simulink library "inp"  (R2021b)
settings: Solver=VariableStepAuto  StartTime=0.0  StopTime=10.0  RelTol=1e-3
undefined symbols (not defined in the file): C_TASK_5MS_S, FALSE, KINP_AcoreReadyToSlp_flg_ovrdflg, KINP_AcoreReadyToSlp_flg_ovrdval, KINP_AllowMovThd_OTA_enum_ovrdflg, KINP_AllowMovThd_OTA_enum_ovrdval, KINP_APSAngleTarget_Deg_ovrdflg, KINP_APSAngleTarget_Deg_ovrdval, KINP_APSDecReq_mps2_ovrdflg, KINP_APSDecReq_mps2_ovrdval, KINP_APSDecReqA_flg_ovrdflg, KINP_APSDecReqA_flg_ovrdval, KINP_APSDFLL_cm_ovrdflg, KINP_APSDFLL_cm_ovrdval, KINP_APSDFLR_cm_ovrdflg, KINP_APSDFLR_cm_ovrdval, KINP_APSDRLL_cm_ovrdflg, KINP_APSDRLL_cm_ovrdval, KINP_APSDRLR_cm_ovrdflg, KINP_APSDRLR_cm_ovrdval, KINP_APSExitCondition_enum_ovrdflg, KINP_APSExitCondition_enum_ovrdval, KINP_APSHWVer_enum_ovrdflg, KINP_APSHWVer_enum_ovrdval, KINP_APSProgressPCT_pct_ovrdflg, KINP_APSProgressPCT_pct_ovrdval, KINP_APSReq_enum_ovrdflg, KINP_APSReq_enum_ovrdval, KINP_APSRQDisplay_enum_ovrdflg, KINP_APSRQDisplay_enum_ovrdval, KINP_APSRqEPASCtrl_flg_ovrdflg, KINP_APSRqEPASCtrl_flg_ovrdval, KINP_APSShiftPosnReq_enum_ovrdval, KINP_APSShiftPosnReq_enum_ovrflg, KINP_APSSpeedCMD_kph_ovrdval, KINP_APSSpeedCMD_kph_ovrflg, KINP_APSStaSystem_enum_ovrdflg, KINP_APSStaSystem_enum_ovrdval, KINP_APSSWVer_enum_ovrdflg, KINP_APSSWVer_enum_ovrdval, KINP_APSVMCReqA_flg_ovrdval, KINP_APSVMCReqA_flg_ovrflg, KINP_APSVRqEPASCtrl_flg_ovrdflg, KINP_APSVRqEPASCtrl_flg_ovrdval, KINP_AuxBattVolmV_mV_ovrdflg, KINP_AuxBattVolmV_mV_ovrdval, KINP_CAASSta_enum_ovrdflg, KINP_CAASSta_enum_ovrdval, KINP_CAASVMCReqA_flg_ovrdval, KINP_CAASVMCReqA_flg_ovrflg, KINP_Chime_enum_ovrdflg, KINP_Chime_enum_ovrdval, KINP_ClearDTCcmd_flg_ovrdflg, KINP_ClearDTCcmd_flg_ovrdval, KINP_EvccAplusPwrUpReq_flg_ovrdflg, KINP_EvccAplusPwrUpReq_flg_ovrdval, KINP_LFID_raw_ovrdval, KINP_LFID_raw_ovrflg, KINP_LRID_raw_ovrdval, KINP_MemOffsetAccX_raw16_ovrdflg ... (+118)
libraries: FVT_lib x503, hcu_lib x1
(part 4 of 16)

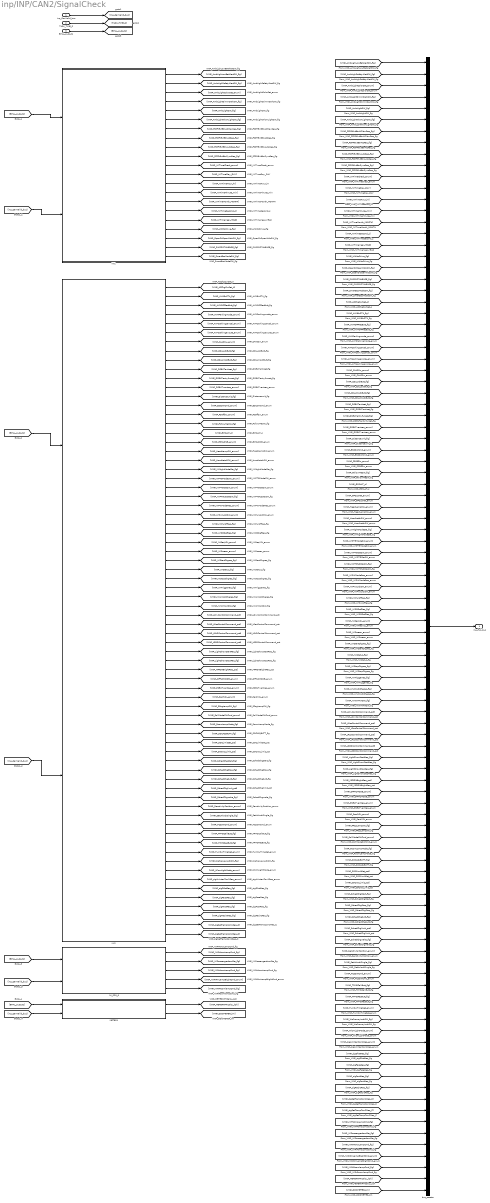
== system inp/INP/CAN2/SignalCheck ==
  inp_CanValid_bus : Inport
  TASK_TIME_S : Inport  Port=2
  BHAL_outputs : Inport  Port=3
  IVI1 : Subsystem
  IVI2 : Subsystem
  IVI_P20_0 : Subsystem
  METER1 : Subsystem
  bus_creator : BusCreator  Inputs=100
  inp_Hal_bus : Outport
  wires:
  inp_CanValid_bus/1 -> [inp_CanValid_bus]
  TASK_TIME_S/1 -> [TASK_TIME_S]
  BHAL_outputs/1 -> [BHAL_outputs]
  [BHAL_outputs] -> IVI1/1(BHAL_outputs)
  [inp_CanValid_bus] -> IVI1/2(inp_CanValid_bus)
  IVI1/1(VINP_AmbLighLowBatAlertSW_flg) -> [VINP_AmbLighLowBatAlertSW_flg]
  IVI1/2(VINP_AmbLighSafetyAlertSW_flg) -> [VINP_AmbLighSafetyAlertSW_flg]
  IVI1/3(VINP_AmbLightColorSet_enum) -> [VINP_AmbLightColorSet_enum]
  IVI1/4(VINP_AmbLightDimInDarkSW_flg) -> [VINP_AmbLightDimInDarkSW_flg]
  IVI1/5(VINP_AmbLightSW_flg) -> [VINP_AmbLightSW_flg]
  IVI1/6(VINP_AmbLightWlcmLightSW_flg) -> [VINP_AmbLightWlcmLightSW_flg]
  IVI1/7(VINP_FCPFrEvtBtnACMaxReq_flg) -> [VINP_FCPFrEvtBtnACMaxReq_flg]
  IVI1/8(VINP_FCPFrEvtBtnACReq_flg) -> [VINP_FCPFrEvtBtnACReq_flg]
  IVI1/9(VINP_FCPFrEvtBtnAutoReq_flg) -> [VINP_FCPFrEvtBtnAutoReq_flg]
  IVI1/10(VINP_FCPFrEvtBtnSyncReq_flg) -> [VINP_FCPFrEvtBtnSyncReq_flg]
  IVI1/11(VINP_IVITimeCheck_enum) -> [VINP_IVITimeCheck_enum]
  IVI1/12(VINP_IVITimeDay_DAY) -> [VINP_IVITimeDay_DAY]
  IVI1/13(VINP_IVITimeHour_hr) -> [VINP_IVITimeHour_hr]
  IVI1/14(VINP_IVITimeMinute_min) -> [VINP_IVITimeMinute_min]
  IVI1/15(VINP_IVITimeMonth_MONTH) -> [VINP_IVITimeMonth_MONTH]
  IVI1/16(VINP_IVITimeSecond_s) -> [VINP_IVITimeSecond_s]
  IVI1/17(VINP_IVITimeYear_YEAR) -> [VINP_IVITimeYear_YEAR]
  IVI1/18(VINP_LINKtoDrive_flg) -> [VINP_LINKtoDrive_flg]
  IVI1/19(VINP_OpenDrOpenWdoSW_flg) -> [VINP_OpenDrOpenWdoSW_flg]
  IVI1/20(VINP_PWCONTINUEUSE_flg) -> [VINP_PWCONTINUEUSE_flg]
  IVI1/21(VINP_SmartEcoModeSW_flg) -> [VINP_SmartEcoModeSW_flg]
  [BHAL_outputs] -> IVI2/1(BHAL_outputs)
  [inp_CanValid_bus] -> IVI2/2(inp_CanValid_bus)
  IVI2/1(VINP_ACChgCurSet_A) -> [VINP_ACChgCurSet_A]
  IVI2/2(VINP_AVMErrSTA_flg) -> [VINP_AVMErrSTA_flg]
  IVI2/3(VINP_AVMOFFRecButt_flg) -> [VINP_AVMOFFRecButt_flg]
  IVI2/4(VINP_AVMParkingmode_enum) -> [VINP_AVMParkingmode_enum]
  IVI2/5(VINP_AVMparkingcancel_enum) -> [VINP_AVMparkingcancel_enum]
  IVI2/6(VINP_AVMparkingexcute_enum) -> [VINP_AVMparkingexcute_enum]
  IVI2/7(VINP_CAASSw_enum) -> [VINP_CAASSw_enum]
  IVI2/8(VINP_CDLLockButt_flg) -> [VINP_CDLLockButt_flg]
  IVI2/9(VINP_CDLUnlockButt_flg) -> [VINP_CDLUnlockButt_flg]
  IVI2/10(VINP_DSEATantiset_flg) -> [VINP_DSEATantiset_flg]
  IVI2/11(VINP_DSEATentryfunset_flg) -> [VINP_DSEATentryfunset_flg]
  IVI2/12(VINP_DSEATventreq_enum) -> [VINP_DSEATventreq_enum]
  IVI2/13(VINP_Distanceunit_flg) -> [VINP_Distanceunit_flg]
  IVI2/14(VINP_ESCSWCmd_enum) -> [VINP_ESCSWCmd_enum]
  IVI2/15(VINP_FSOffSw_enum) -> [VINP_FSOffSw_enum]
  IVI2/16(VINP_FollowMeSW_flg) -> [VINP_FollowMeSW_flg]
  IVI2/17(VINP_GPSLAT_s) -> [VINP_GPSLAT_s]
  IVI2/18(VINP_GPSLONG_enum) -> [VINP_GPSLONG_enum]
  IVI2/19(VINP_HeadLampSW_enum) -> [VINP_HeadLampSW_enum]
  IVI2/20(VINP_HoodLatchSW_enum) -> [VINP_HoodLatchSW_enum]
  IVI2/21(VINP_IVINightModeSta_flg) -> [VINP_IVINightModeSta_flg]
  IVI2/22(VINP_IVIPTGModeSW_enum) -> [VINP_IVIPTGModeSW_enum]
  IVI2/23(VINP_IVIPTGStaSW_enum) -> [VINP_IVIPTGStaSW_enum]
  IVI2/24(VINP_IVIPTGUSStaSW_flg) -> [VINP_IVIPTGUSStaSW_flg]
  IVI2/25(VINP_IVIPWModeReq_enum) -> [VINP_IVIPWModeReq_enum]
  IVI2/26(VINP_IVIPwrLockSW_enum) -> [VINP_IVIPwrLockSW_enum]
  IVI2/27(VINP_IVIPwroffreq_flg) -> [VINP_IVIPwroffreq_flg]
  IVI2/28(VINP_IVIRRDefReq_flg) -> [VINP_IVIRRDefReq_flg]
  IVI2/29(VINP_IVIReqV2L_enum) -> [VINP_IVIReqV2L_enum]
  IVI2/30(VINP_IVIScreen_enum) -> [VINP_IVIScreen_enum]
  IVI2/31(VINP_IVIStartChgreq_flg) -> [VINP_IVIStartChgreq_flg]
  IVI2/32(VINP_IVIStatus_flg) -> [VINP_IVIStatus_flg]
  IVI2/33(VINP_IVIStopChgreq_flg) -> [VINP_IVIStopChgreq_flg]
  IVI2/34(VINP_IVITriggerreq_flg) -> [VINP_IVITriggerreq_flg]
  IVI2/35(VINP_IVIUnlockChgreq_flg) -> [VINP_IVIUnlockChgreq_flg]
  IVI2/36(VINP_IVIWIMAINSW_flg) -> [VINP_IVIWIMAINSW_flg]
  IVI2/37(VINP_LDrvControlCommand_pct) -> [VINP_LDrvControlCommand_pct]
  IVI2/38(VINP_LPasControlCommand_pct) -> [VINP_LPasControlCommand_pct]
  IVI2/39(VINP_LRLDControlCommand_pct) -> [VINP_LRLDControlCommand_pct]
  IVI2/40(VINP_LRRDControlCommand_pct) -> [VINP_LRRDControlCommand_pct]
  IVI2/41(VINP_LightShowStartReq_flg) -> [VINP_LightShowStartReq_flg]
  IVI2/42(VINP_LightShowStopReq_flg) -> [VINP_LightShowStopReq_flg]
  IVI2/43(VINP_MFRDNBrightReq_pct) -> [VINP_MFRDNBrightReq_pct]
  IVI2/44(VINP_OFFACMODE_enum) -> [VINP_OFFACMODE_enum]
  IVI2/45(VINP_PSEATventreq_enum) -> [VINP_PSEATventreq_enum]
  IVI2/46(VINP_PerdV2L_enum) -> [VINP_PerdV2L_enum]
  IVI2/47(VINP_RFogLampSW_flg) -> [VINP_RFogLampSW_flg]
  IVI2/48(VINP_RollModeSWCmd_enum) -> [VINP_RollModeSWCmd_enum]
  IVI2/49(VINP_RoomLampMode_flg) -> [VINP_RoomLampMode_flg]
  IVI2/50(VINP_SOCADJBUTT_flg) -> [VINP_SOCADJBUTT_flg]
  IVI2/51(VINP_SOCLimitSet_pct) -> [VINP_SOCLimitSet_pct]
  IVI2/52(VINP_SOCV2LLimit_pct) -> [VINP_SOCV2LLimit_pct]
  IVI2/53(VINP_SchedChgStart_flg) -> [VINP_SchedChgStart_flg]
  IVI2/54(VINP_SchedChgStop_flg) -> [VINP_SchedChgStop_flg]
  IVI2/55(VINP_SchedChgbutt_flg) -> [VINP_SchedChgbutt_flg]
  IVI2/56(VINP_SchedChglimit_pct) -> [VINP_SchedChglimit_pct]
  IVI2/57(VINP_SchedChgwake_flg) -> [VINP_SchedChgwake_flg]
  IVI2/58(VINP_SenstivityPosition_enum) -> [VINP_SenstivityPosition_enum]
  IVI2/59(VINP_SetUnlockSingle_flg) -> [VINP_SetUnlockSingle_flg]
  IVI2/60(VINP_TCSSWCmd_enum) -> [VINP_TCSSWCmd_enum]
  IVI2/61(VINP_TPMSCaliButt_flg) -> [VINP_TPMSCaliButt_flg]
  IVI2/62(VINP_TPMSResButt_flg) -> [VINP_TPMSResButt_flg]
  IVI2/63(VINP_TurnSwTimeSet_enum) -> [VINP_TurnSwTimeSet_enum]
  IVI2/64(VINP_WalkawayLockSW_flg) -> [VINP_WalkawayLockSW_flg]
  IVI2/65(VINP_WlcmLightMode_enum) -> [VINP_WlcmLightMode_enum]
  IVI2/66(VINP_sigAirIntenZon1Req_enum) -> [VINP_sigAirIntenZon1Req_enum]
  IVI2/67(VINP_sigDfrstReq_flg) -> [VINP_sigDfrstReq_flg]
  IVI2/68(VINP_sigFaceReq_flg) -> [VINP_sigFaceReq_flg]
  IVI2/69(VINP_sigFootReq_flg) -> [VINP_sigFootReq_flg]
  IVI2/70(VINP_sigRecircReq_flg) -> [VINP_sigRecircReq_flg]
  IVI2/71(VINP_sigSetTempZon1Req_C) -> [VINP_sigSetTempZon1Req_C]
  IVI2/72(VINP_sigSetTempZon2Req_C) -> [VINP_sigSetTempZon2Req_C]
  [BHAL_outputs] -> IVI_P20_0/1(BHAL_outputs)
  [inp_CanValid_bus] -> IVI_P20_0/2(inp_CanValid_bus)
  IVI_P20_0/1(VINP_IVIFrAtmoLampCmd_flg) -> [VINP_IVIFrAtmoLampCmd_flg]
  IVI_P20_0/2(VINP_IVIPassengerdoorSta_flg) -> [VINP_IVIPassengerdoorSta_flg]
  IVI_P20_0/3(VINP_IVIRrAtmoLampCmd_flg) -> [VINP_IVIRrAtmoLampCmd_flg]
  IVI_P20_0/4(VINP_IVIRrRmLampBrightCmd_enum) -> [VINP_IVIRrRmLampBrightCmd_enum]
  IVI_P20_0/5(VINP_IVIRrRoomlampCmd_flg) -> [VINP_IVIRrRoomlampCmd_flg]
  [BHAL_outputs] -> METER1/1(BHAL_outputs)
  [inp_CanValid_bus] -> METER1/2(inp_CanValid_bus)
  METER1/1(VINP_METERKPHCalcu_kph) -> [VINP_METERKPHCalcu_kph]
  METER1/2(VINP_ODOMETER_km) -> [VINP_ODOMETER_km]
  bus_creator/1 -> inp_Hal_bus/1
  [VINP_AmbLighLowBatAlertSW_flg] -> bus_creator/1
  [VINP_AmbLighSafetyAlertSW_flg] -> bus_creator/2
  [VINP_AmbLightColorSet_enum] -> bus_creator/3
  [VINP_AmbLightDimInDarkSW_flg] -> bus_creator/4
  [VINP_AmbLightSW_flg] -> bus_creator/5
  [VINP_AmbLightWlcmLightSW_flg] -> bus_creator/6
  [VINP_FCPFrEvtBtnACMaxReq_flg] -> bus_creator/7
  [VINP_FCPFrEvtBtnACReq_flg] -> bus_creator/8
  [VINP_FCPFrEvtBtnAutoReq_flg] -> bus_creator/9
  [VINP_FCPFrEvtBtnSyncReq_flg] -> bus_creator/10
  [VINP_IVITimeCheck_enum] -> bus_creator/11
  [VINP_IVITimeDay_DAY] -> bus_creator/12
  [VINP_IVITimeHour_hr] -> bus_creator/13
  [VINP_IVITimeMinute_min] -> bus_creator/14
  [VINP_IVITimeMonth_MONTH] -> bus_creator/15
  [VINP_IVITimeSecond_s] -> bus_creator/16
  [VINP_IVITimeYear_YEAR] -> bus_creator/17
  [VINP_LINKtoDrive_flg] -> bus_creator/18
  [VINP_OpenDrOpenWdoSW_flg] -> bus_creator/19
  [VINP_PWCONTINUEUSE_flg] -> bus_creator/20
  [VINP_SmartEcoModeSW_flg] -> bus_creator/21
  [VINP_ACChgCurSet_A] -> bus_creator/22
  [VINP_AVMErrSTA_flg] -> bus_creator/23
  [VINP_AVMOFFRecButt_flg] -> bus_creator/24
  [VINP_AVMParkingmode_enum] -> bus_creator/25
  [VINP_AVMparkingcancel_enum] -> bus_creator/26
  [VINP_AVMparkingexcute_enum] -> bus_creator/27
  [VINP_CAASSw_enum] -> bus_creator/28
  [VINP_CDLLockButt_flg] -> bus_creator/29
  [VINP_CDLUnlockButt_flg] -> bus_creator/30
  [VINP_DSEATantiset_flg] -> bus_creator/31
  [VINP_DSEATentryfunset_flg] -> bus_creator/32
  [VINP_DSEATventreq_enum] -> bus_creator/33
  [VINP_Distanceunit_flg] -> bus_creator/34
  [VINP_ESCSWCmd_enum] -> bus_creator/35
  [VINP_FSOffSw_enum] -> bus_creator/36
  [VINP_FollowMeSW_flg] -> bus_creator/37
  [VINP_GPSLAT_s] -> bus_creator/38
  [VINP_GPSLONG_enum] -> bus_creator/39
  [VINP_HeadLampSW_enum] -> bus_creator/40
  [VINP_HoodLatchSW_enum] -> bus_creator/41
  [VINP_IVINightModeSta_flg] -> bus_creator/42
  [VINP_IVIPTGModeSW_enum] -> bus_creator/43
  [VINP_IVIPTGStaSW_enum] -> bus_creator/44
  [VINP_IVIPTGUSStaSW_flg] -> bus_creator/45
  [VINP_IVIPWModeReq_enum] -> bus_creator/46
  [VINP_IVIPwrLockSW_enum] -> bus_creator/47
  [VINP_IVIPwroffreq_flg] -> bus_creator/48
  [VINP_IVIRRDefReq_flg] -> bus_creator/49
  [VINP_IVIReqV2L_enum] -> bus_creator/50
  [VINP_IVIScreen_enum] -> bus_creator/51
  [VINP_IVIStartChgreq_flg] -> bus_creator/52
  [VINP_IVIStatus_flg] -> bus_creator/53
  [VINP_IVIStopChgreq_flg] -> bus_creator/54
  [VINP_IVITriggerreq_flg] -> bus_creator/55
  [VINP_IVIUnlockChgreq_flg] -> bus_creator/56
  [VINP_IVIWIMAINSW_flg] -> bus_creator/57
  [VINP_LDrvControlCommand_pct] -> bus_creator/58
  [VINP_LPasControlCommand_pct] -> bus_creator/59
  [VINP_LRLDControlCommand_pct] -> bus_creator/60
  [VINP_LRRDControlCommand_pct] -> bus_creator/61
  [VINP_LightShowStartReq_flg] -> bus_creator/62
  [VINP_LightShowStopReq_flg] -> bus_creator/63
  [VINP_MFRDNBrightReq_pct] -> bus_creator/64
  [VINP_OFFACMODE_enum] -> bus_creator/65
  [VINP_PSEATventreq_enum] -> bus_creator/66
  [VINP_PerdV2L_enum] -> bus_creator/67
  [VINP_RFogLampSW_flg] -> bus_creator/68
  [VINP_RollModeSWCmd_enum] -> bus_creator/69
  [VINP_RoomLampMode_flg] -> bus_creator/70
  [VINP_SOCADJBUTT_flg] -> bus_creator/71
  [VINP_SOCLimitSet_pct] -> bus_creator/72
  [VINP_SOCV2LLimit_pct] -> bus_creator/73
  [VINP_SchedChgStart_flg] -> bus_creator/74
  [VINP_SchedChgStop_flg] -> bus_creator/75
  [VINP_SchedChgbutt_flg] -> bus_creator/76
  [VINP_SchedChglimit_pct] -> bus_creator/77
  [VINP_SchedChgwake_flg] -> bus_creator/78
  [VINP_SenstivityPosition_enum] -> bus_creator/79
  [VINP_SetUnlockSingle_flg] -> bus_creator/80
  [VINP_TCSSWCmd_enum] -> bus_creator/81
  [VINP_TPMSCaliButt_flg] -> bus_creator/82
  [VINP_TPMSResButt_flg] -> bus_creator/83
  [VINP_TurnSwTimeSet_enum] -> bus_creator/84
  [VINP_WalkawayLockSW_flg] -> bus_creator/85
  [VINP_WlcmLightMode_enum] -> bus_creator/86
  [VINP_sigAirIntenZon1Req_enum] -> bus_creator/87
  [VINP_sigDfrstReq_flg] -> bus_creator/88
  [VINP_sigFaceReq_flg] -> bus_creator/89
  [VINP_sigFootReq_flg] -> bus_creator/90
  [VINP_sigRecircReq_flg] -> bus_creator/91
  [VINP_sigSetTempZon1Req_C] -> bus_creator/92
  [VINP_sigSetTempZon2Req_C] -> bus_creator/93
  [VINP_IVIFrAtmoLampCmd_flg] -> bus_creator/94
  [VINP_IVIPassengerdoorSta_flg] -> bus_creator/95
  [VINP_IVIRrAtmoLampCmd_flg] -> bus_creator/96
  [VINP_IVIRrRmLampBrightCmd_enum] -> bus_creator/97
  [VINP_IVIRrRoomlampCmd_flg] -> bus_creator/98
  [VINP_METERKPHCalcu_kph] -> bus_creator/99
  [VINP_ODOMETER_km] -> bus_creator/100

== system inp/INP/CAN3/CommunicationCheck ==
  BHAL_outputs : Inport
  CANMsgInvalidBMS1 : FVT_lib/inp/CAN_Msg_Validity_Process_template  SystemSampleTime=-1  VariantActivationTime=update diagram  Latency=0  AutoFrameSizeCalculation=off
      link override ovrdflg: Value=KINP_CANMsgInvalidBMS1_flg_ovrdflg
      link override ovrdval: Value=KINP_CANMsgInvalidBMS1_flg_ovrdval
  CANMsgInvalidBMS3 : FVT_lib/inp/CAN_Msg_Validity_Process_template  SystemSampleTime=-1  VariantActivationTime=update diagram  Latency=0  AutoFrameSizeCalculation=off
      link override ovrdflg: Value=KINP_CANMsgInvalidBMS3_flg_ovrdflg
      link override ovrdval: Value=KINP_CANMsgInvalidBMS3_flg_ovrdval
  CANMsgInvalidBMS4 : FVT_lib/inp/CAN_Msg_Validity_Process_template  SystemSampleTime=-1  VariantActivationTime=update diagram  Latency=0  AutoFrameSizeCalculation=off
      link override ovrdflg: Value=KINP_CANMsgInvalidBMS4_flg_ovrdflg
      link override ovrdval: Value=KINP_CANMsgInvalidBMS4_flg_ovrdval
  CANMsgInvalidBMS5 : FVT_lib/inp/CAN_Msg_Validity_Process_template  SystemSampleTime=-1  VariantActivationTime=update diagram  Latency=0  AutoFrameSizeCalculation=off
      link override ovrdflg: Value=KINP_CANMsgInvalidBMS5_flg_ovrdflg
      link override ovrdval: Value=KINP_CANMsgInvalidBMS5_flg_ovrdval
  CANMsgInvalidBMS6 : FVT_lib/inp/CAN_Msg_Validity_Process_template  SystemSampleTime=-1  VariantActivationTime=update diagram  Latency=0  AutoFrameSizeCalculation=off
      link override ovrdflg: Value=KINP_CANMsgInvalidBMS6_flg_ovrdflg
      link override ovrdval: Value=KINP_CANMsgInvalidBMS6_flg_ovrdval
  CANMsgInvalidBMS8 : FVT_lib/inp/CAN_Msg_Validity_Process_template  SystemSampleTime=-1  VariantActivationTime=update diagram  Latency=0  AutoFrameSizeCalculation=off
      link override ovrdflg: Value=KINP_CANMsgInvalidBMS8_flg_ovrdflg
      link override ovrdval: Value=KINP_CANMsgInvalidBMS8_flg_ovrdval
  CANMsgInvalidCCU1 : FVT_lib/inp/CAN_Msg_Validity_Process_template  SystemSampleTime=-1  VariantActivationTime=update diagram  Latency=0  AutoFrameSizeCalculation=off
      link override ovrdflg: Value=KINP_CANMsgInvalidCCU1_flg_ovrdflg
      link override ovrdval: Value=KINP_CANMsgInvalidCCU1_flg_ovrdval
  CANMsgInvalidCCU2 : FVT_lib/inp/CAN_Msg_Validity_Process_template  SystemSampleTime=-1  VariantActivationTime=update diagram  Latency=0  AutoFrameSizeCalculation=off
      link override ovrdflg: Value=KINP_CANMsgInvalidCCU2_flg_ovrdflg
      link override ovrdval: Value=KINP_CANMsgInvalidCCU2_flg_ovrdval
  CANMsgInvalidMCUBR1 : FVT_lib/inp/CAN_Msg_Validity_Process_template  SystemSampleTime=-1  VariantActivationTime=update diagram  Latency=0  AutoFrameSizeCalculation=off
      link override ovrdflg: Value=KINP_CANMsgInvalidMCUBR1_flg_ovrdflg
      link override ovrdval: Value=KINP_CANMsgInvalidMCUBR1_flg_ovrdval
  CANMsgInvalidMCUBR2 : FVT_lib/inp/CAN_Msg_Validity_Process_template  SystemSampleTime=-1  VariantActivationTime=update diagram  Latency=0  AutoFrameSizeCalculation=off
      link override ovrdflg: Value=KINP_CANMsgInvalidMCUBR2_flg_ovrdflg
      link override ovrdval: Value=KINP_CANMsgInvalidMCUBR2_flg_ovrdval
  CANMsgInvalidShifter1 : FVT_lib/inp/CAN_Msg_Validity_Process_template  SystemSampleTime=-1  VariantActivationTime=update diagram  Latency=0  AutoFrameSizeCalculation=off
      link override ovrdflg: Value=KINP_CANMsgInvalidShifter1_flg_ovrdflg
      link override ovrdval: Value=KINP_CANMsgInvalidShifter1_flg_ovrdval
  bus_creator : BusCreator  Inputs=11
  bus_selector : BusSelector  OutputSignals=VHAL_CANMsgInvalidBMS1_flg,VHAL_CANMsgInvalidBMS3_flg,VHAL_CANMsgInvalidBMS4_flg,VHAL_CANMsgInvalidBMS5_flg,VHAL_CANMsgInvalidBMS6_flg,VHAL_CANMsgInvalidBMS8_flg,VHAL_CANMsgInvalidCCU1_flg,VHAL_CANMsgInvalidCCU2_flg,VHAL_CANMsgInvalidMCUBR1_flg,VHAL_CANMsgInvalidMCUBR2_flg,VHAL_CANMsgInvalidShifter1_flg
  not{1..11} (11 alike) : Logic  Operator=NOT  AllPortsSameDT=off  OutDataTypeStr=boolean
  inp_CanValid_bus : Outport
  wires:
  BHAL_outputs/1 -> [BHAL_outputs]
  bus_selector/1 -> CANMsgInvalidBMS1/1  "<VHAL_CANMsgInvalidBMS1_flg>"
  CANMsgInvalidBMS1/1 -> not1/1
  not1/1 -> bus_creator/1  "VINP_CANMsgValidBMS1_flg"
  bus_selector/2 -> CANMsgInvalidBMS3/1  "<VHAL_CANMsgInvalidBMS3_flg>"
  CANMsgInvalidBMS3/1 -> not2/1
  not2/1 -> bus_creator/2  "VINP_CANMsgValidBMS3_flg"
  bus_selector/3 -> CANMsgInvalidBMS4/1  "<VHAL_CANMsgInvalidBMS4_flg>"
  CANMsgInvalidBMS4/1 -> not3/1
  not3/1 -> bus_creator/3  "VINP_CANMsgValidBMS4_flg"
  bus_selector/4 -> CANMsgInvalidBMS5/1  "<VHAL_CANMsgInvalidBMS5_flg>"
  CANMsgInvalidBMS5/1 -> not4/1
  not4/1 -> bus_creator/4  "VINP_CANMsgValidBMS5_flg"
  bus_selector/5 -> CANMsgInvalidBMS6/1  "<VHAL_CANMsgInvalidBMS6_flg>"
  CANMsgInvalidBMS6/1 -> not5/1
  not5/1 -> bus_creator/5  "VINP_CANMsgValidBMS6_flg"
  bus_selector/6 -> CANMsgInvalidBMS8/1  "<VHAL_CANMsgInvalidBMS8_flg>"
  CANMsgInvalidBMS8/1 -> not6/1
  not6/1 -> bus_creator/6  "VINP_CANMsgValidBMS8_flg"
  bus_selector/7 -> CANMsgInvalidCCU1/1  "<VHAL_CANMsgInvalidCCU1_flg>"
  CANMsgInvalidCCU1/1 -> not7/1
  not7/1 -> bus_creator/7  "VINP_CANMsgValidCCU1_flg"
  bus_selector/8 -> CANMsgInvalidCCU2/1  "<VHAL_CANMsgInvalidCCU2_flg>"
  CANMsgInvalidCCU2/1 -> not8/1
  not8/1 -> bus_creator/8  "VINP_CANMsgValidCCU2_flg"
  bus_selector/9 -> CANMsgInvalidMCUBR1/1  "<VHAL_CANMsgInvalidMCUBR1_flg>"
  CANMsgInvalidMCUBR1/1 -> not9/1
  not9/1 -> bus_creator/9  "VINP_CANMsgValidMCUBR1_flg"
  bus_selector/10 -> CANMsgInvalidMCUBR2/1  "<VHAL_CANMsgInvalidMCUBR2_flg>"
  CANMsgInvalidMCUBR2/1 -> not10/1
  not10/1 -> bus_creator/10  "VINP_CANMsgValidMCUBR2_flg"
  bus_selector/11 -> CANMsgInvalidShifter1/1  "<VHAL_CANMsgInvalidShifter1_flg>"
  CANMsgInvalidShifter1/1 -> not11/1
  not11/1 -> bus_creator/11  "VINP_CANMsgValidShifter1_flg"
  [BHAL_outputs] -> bus_selector/1
  bus_creator/1 -> inp_CanValid_bus/1

== system inp/INP/CAN3/CreateBus ==
  inp_CanValid_bus : Inport
  inp_Hal_bus : Inport  Port=2
  UnitConverter_{1..11,23,32,52..60,65..67,71,84,87,89,93,95..96,102..104,111..112,114..116} (40 alike) : DataTypeConversion  OutDataTypeStr=boolean
  UnitConverter_{12..13,42..45,50..51,61..64,68..70,72..75,80,83,85..86,88,94,98..101,106,113,117,126..129,134..139} (42 alike) : DataTypeConversion  OutDataTypeStr=uint8
  UnitConverter_{14..22,24..31,33..41,46..49,76..79,81..82,90..92,97,105,107..110,118..125,130..131} (55 alike) : DataTypeConversion  OutDataTypeStr=single
  UnitConverter_132 : DataTypeConversion  OutDataTypeStr=uint16
  UnitConverter_133 : DataTypeConversion  OutDataTypeStr=uint16
  bus_creator : BusCreator  Inputs=139
  bus_selector : BusSelector  OutputSignals=VINP_CANMsgValidBMS1_flg,VINP_CANMsgValidBMS3_flg,VINP_CANMsgValidBMS4_flg,VINP_CANMsgValidBMS5_flg,VINP_CANMsgValidBMS6_flg,VINP_CANMsgValidBMS8_flg,VINP_CANMsgValidCCU1_flg,VINP_CANMsgValidCCU2_flg,VINP_CANMsgValidMCUBR1_flg,VINP_CANMsgValidMCUBR2_flg,VINP_CANMsgValidShifter1_flg
  bus_selector_1 : BusSelector  OutputSignals=VINP_BMSChckSum1_enum,VINP_BMSRolCnct1_enum,VINP_HVBPwrAvailChrg_kW,VINP_HVBPwrAvailChrg30_kW,VINP_HVBPwrAvailChrg60_kW,VINP_HVBPwrAvailDchrg_kW,VINP_HVBPwrAvailDchrg30_kW,VINP_HVBPwrAvailDchrg60_kW,VINP_HVBattCurr_A,VINP_HVBattVolt_V,VINP_ACChrgCurrDis_A,VINP_FireDetErr_flg,VINP_HVBChrgPwr_kWh,VINP_HVBChrgPwrTotal_kWh,VINP_HVBDrvPwr_kWh,VINP_HVBDrvPwrTotal_kWh,VINP_HVBFullChrgPwr_kWh,VINP_HVBIsoImpedenceN_Megaohm,VINP_HVBIsoImpedenceP_Megaohm,VINP_HVBSOH_pct,VINP_HVBattErr_flg,VINP_HVBattPackVolt_V,VINP_HVBattSOC_pct,VINP_HVBattSOCDis_pct,VINP_RemainChrgTime_min,VINP_CellTempAvg_C,VINP_HVBCellVoltMax_mV,VINP_HVBCellVoltMin_mV,VINP_HVBMTempMax_C,VINP_HVBMTempMin_C,VINP_MaxCellTempNum_enum,VINP_MaxCellVoltNum_enum,VINP_MinCellTempNum_enum,VINP_MinCellVoltNum_enum,VINP_HVInVolt_V,VINP_LVBattDet12V_V,VINP_OBCDCCurLm_A,VINP_OBCDCVoltLm_V,VINP_BMSChckSum_enum,VINP_BMSRolCnct_enum,VINP_BMSREADY_flg,VINP_BMSWarn1_flg,VINP_BMSWarn2_flg,VINP_BMSWarn3_flg,VINP_BMSWarn4_flg,VINP_BMSWarn5_flg,VINP_BMSWarn6_flg,VINP_BMSWarn7_flg,VINP_BMSWarn8_flg,VINP_ChrgPlugSta_enum,VINP_DisChrgPlugErr_enum,VINP_ExtChrgSta_enum,VINP_HVBChrgErr_enum,VINP_HVBContactorSta_flg,VINP_HVBHVILErr_flg,VINP_HVBOvrTempErr_flg,VINP_HVBOvrTempWarn_enum,VINP_HVBPreheatPrecoolSta_enum,VINP_HVBattReady4Pre_enum,VINP_HVILSta_flg,VINP_V2LSta_enum,VINP_MainRlyNegSta_enum,VINP_MainRlyPosSta_enum,VINP_CSCCU1_enum,VINP_DCDCAuxCur_A,VINP_DCDCAuxVolt_V,VINP_DCDCHVCur_A,VINP_DCDCInVoltInf_V,VINP_DCDCPreCompleted_enum,VINP_OBCDCCurrInf_A,VINP_OBCDCVoltInf_V,VINP_OBCPreCompleted_enum,VINP_OBCWakeup4Plugin_flg,VINP_RCCCU1_enum,VINP_CSCCU2_enum,VINP_DCDCEnaSta_flg,VINP_DCDCFaultSta_enum,VINP_DCDCReady4Pre_flg,VINP_DCDCTemp_C,VINP_OBCACCurrInf_A,VINP_OBCACVoltInf_V,VINP_OBCEnaSta_flg,VINP_OBCFaultSta_enum,VINP_OBCPluginSta_flg,VINP_OBCReady4Pre_flg,VINP_OBCTemp_C,VINP_OBCV2LSta_enum,VINP_OBCACCurLim_enum,VINP_RCCCU2_enum,VINP_MCUWarnR_enum,VINP_RrActvDmpDisabSta_flg,VINP_RrEDUDrtSta_flg,VINP_RrEDUOpratingSta_flg,VINP_RrEDURealTMTq_Nm,VINP_RrEDURotateDirction_enum,VINP_RrEDUTqReqFbk_Nm,VINP_RrMCUBAT_V,VINP_RrMCUDCBusCurr_A,VINP_RrMCUDCBusVolt_V,VINP_RrMCUDischrgSta_flg,VINP_RrMCUEnaSta_flg,VINP_RrMCUErr_enum,VINP_RrMCUIGNsta_flg,VINP_RrMCUReady_flg,VINP_RrMCUReady4Pre_flg,VINP_RrMCUSysSta_enum,VINP_RrMCUTemp_C,VINP_RrMotorAvailTq_Nm,VINP_RrRegenAvailTq_Nm,VINP_RrTMSpd_rpm,VINP_RrTMTemp_C,VINP_RrTMid_A,VINP_RrTMiq_A,VINP_RrCoolanttempReq_cnt,VINP_RrFailcode1_enum,VINP_RrFailcode2_enum,VINP_RrFailcodehistory1_enum,VINP_RrFailcodehistory2_enum,VINP_RrLLCTemp_C,VINP_RrLLCflowReq_Lpmin,VINP_RrMCU3HWVer_enum,VINP_RrMCU3SWVer_enum,VINP_RrMCUTempWarn_enum,VINP_RrTMTempWarn_enum,VINP_ShifterCRC8_enum,VINP_ShifterFailsta_enum,VINP_ShifterHandleCmd_enum,VINP_ShifterRC_enum
  BINP_outputs : Outport
  wires:
  inp_CanValid_bus/1 -> [inp_CanValid_bus]
  inp_Hal_bus/1 -> [inp_Hal_bus]
  bus_selector/1 -> UnitConverter_1/1  "<VINP_CANMsgValidBMS1_flg>"
  UnitConverter_1/1 -> bus_creator/1  "VINP_CANMsgValidBMS1_flg"
  bus_selector/2 -> UnitConverter_2/1  "<VINP_CANMsgValidBMS3_flg>"
  UnitConverter_2/1 -> bus_creator/2  "VINP_CANMsgValidBMS3_flg"
  bus_selector/3 -> UnitConverter_3/1  "<VINP_CANMsgValidBMS4_flg>"
  UnitConverter_3/1 -> bus_creator/3  "VINP_CANMsgValidBMS4_flg"
  bus_selector/4 -> UnitConverter_4/1  "<VINP_CANMsgValidBMS5_flg>"
  UnitConverter_4/1 -> bus_creator/4  "VINP_CANMsgValidBMS5_flg"
  bus_selector/5 -> UnitConverter_5/1  "<VINP_CANMsgValidBMS6_flg>"
  UnitConverter_5/1 -> bus_creator/5  "VINP_CANMsgValidBMS6_flg"
  bus_selector/6 -> UnitConverter_6/1  "<VINP_CANMsgValidBMS8_flg>"
  UnitConverter_6/1 -> bus_creator/6  "VINP_CANMsgValidBMS8_flg"
  bus_selector/7 -> UnitConverter_7/1  "<VINP_CANMsgValidCCU1_flg>"
  UnitConverter_7/1 -> bus_creator/7  "VINP_CANMsgValidCCU1_flg"
  bus_selector/8 -> UnitConverter_8/1  "<VINP_CANMsgValidCCU2_flg>"
  UnitConverter_8/1 -> bus_creator/8  "VINP_CANMsgValidCCU2_flg"
  bus_selector/9 -> UnitConverter_9/1  "<VINP_CANMsgValidMCUBR1_flg>"
  UnitConverter_9/1 -> bus_creator/9  "VINP_CANMsgValidMCUBR1_flg"
  bus_selector/10 -> UnitConverter_10/1  "<VINP_CANMsgValidMCUBR2_flg>"
  UnitConverter_10/1 -> bus_creator/10  "VINP_CANMsgValidMCUBR2_flg"
  bus_selector/11 -> UnitConverter_11/1  "<VINP_CANMsgValidShifter1_flg>"
  UnitConverter_11/1 -> bus_creator/11  "VINP_CANMsgValidShifter1_flg"
  bus_selector_1/1 -> UnitConverter_12/1  "<VINP_BMSChckSum1_enum>"
  UnitConverter_12/1 -> bus_creator/12  "VINP_BMSChckSum1_enum"
  bus_selector_1/2 -> UnitConverter_13/1  "<VINP_BMSRolCnct1_enum>"
  UnitConverter_13/1 -> bus_creator/13  "VINP_BMSRolCnct1_enum"
  bus_selector_1/3 -> UnitConverter_14/1  "<VINP_HVBPwrAvailChrg_kW>"
  UnitConverter_14/1 -> bus_creator/14  "VINP_HVBPwrAvailChrg_kW"
  bus_selector_1/4 -> UnitConverter_15/1  "<VINP_HVBPwrAvailChrg30_kW>"
  UnitConverter_15/1 -> bus_creator/15  "VINP_HVBPwrAvailChrg30_kW"
  bus_selector_1/5 -> UnitConverter_16/1  "<VINP_HVBPwrAvailChrg60_kW>"
  UnitConverter_16/1 -> bus_creator/16  "VINP_HVBPwrAvailChrg60_kW"
  bus_selector_1/6 -> UnitConverter_17/1  "<VINP_HVBPwrAvailDchrg_kW>"
  UnitConverter_17/1 -> bus_creator/17  "VINP_HVBPwrAvailDchrg_kW"
  bus_selector_1/7 -> UnitConverter_18/1  "<VINP_HVBPwrAvailDchrg30_kW>"
  UnitConverter_18/1 -> bus_creator/18  "VINP_HVBPwrAvailDchrg30_kW"
  bus_selector_1/8 -> UnitConverter_19/1  "<VINP_HVBPwrAvailDchrg60_kW>"
  UnitConverter_19/1 -> bus_creator/19  "VINP_HVBPwrAvailDchrg60_kW"
  bus_selector_1/9 -> UnitConverter_20/1  "<VINP_HVBattCurr_A>"
  UnitConverter_20/1 -> bus_creator/20  "VINP_HVBattCurr_A"
  bus_selector_1/10 -> UnitConverter_21/1  "<VINP_HVBattVolt_V>"
  UnitConverter_21/1 -> bus_creator/21  "VINP_HVBattVolt_V"
  bus_selector_1/11 -> UnitConverter_22/1  "<VINP_ACChrgCurrDis_A>"
  UnitConverter_22/1 -> bus_creator/22  "VINP_ACChrgCurrDis_A"
  bus_selector_1/12 -> UnitConverter_23/1  "<VINP_FireDetErr_flg>"
  UnitConverter_23/1 -> bus_creator/23  "VINP_FireDetErr_flg"
  bus_selector_1/13 -> UnitConverter_24/1  "<VINP_HVBChrgPwr_kWh>"
  UnitConverter_24/1 -> bus_creator/24  "VINP_HVBChrgPwr_kWh"
  bus_selector_1/14 -> UnitConverter_25/1  "<VINP_HVBChrgPwrTotal_kWh>"
  UnitConverter_25/1 -> bus_creator/25  "VINP_HVBChrgPwrTotal_kWh"
  bus_selector_1/15 -> UnitConverter_26/1  "<VINP_HVBDrvPwr_kWh>"
  UnitConverter_26/1 -> bus_creator/26  "VINP_HVBDrvPwr_kWh"
  bus_selector_1/16 -> UnitConverter_27/1  "<VINP_HVBDrvPwrTotal_kWh>"
  UnitConverter_27/1 -> bus_creator/27  "VINP_HVBDrvPwrTotal_kWh"
  bus_selector_1/17 -> UnitConverter_28/1  "<VINP_HVBFullChrgPwr_kWh>"
  UnitConverter_28/1 -> bus_creator/28  "VINP_HVBFullChrgPwr_kWh"
  bus_selector_1/18 -> UnitConverter_29/1  "<VINP_HVBIsoImpedenceN_Megaohm>"
  UnitConverter_29/1 -> bus_creator/29  "VINP_HVBIsoImpedenceN_Megaohm"
  bus_selector_1/19 -> UnitConverter_30/1  "<VINP_HVBIsoImpedenceP_Megaohm>"
  UnitConverter_30/1 -> bus_creator/30  "VINP_HVBIsoImpedenceP_Megaohm"
  bus_selector_1/20 -> UnitConverter_31/1  "<VINP_HVBSOH_pct>"
  UnitConverter_31/1 -> bus_creator/31  "VINP_HVBSOH_pct"
  bus_selector_1/21 -> UnitConverter_32/1  "<VINP_HVBattErr_flg>"
  UnitConverter_32/1 -> bus_creator/32  "VINP_HVBattErr_flg"
  bus_selector_1/22 -> UnitConverter_33/1  "<VINP_HVBattPackVolt_V>"
  UnitConverter_33/1 -> bus_creator/33  "VINP_HVBattPackVolt_V"
  bus_selector_1/23 -> UnitConverter_34/1  "<VINP_HVBattSOC_pct>"
  UnitConverter_34/1 -> bus_creator/34  "VINP_HVBattSOC_pct"
  bus_selector_1/24 -> UnitConverter_35/1  "<VINP_HVBattSOCDis_pct>"
  UnitConverter_35/1 -> bus_creator/35  "VINP_HVBattSOCDis_pct"
  bus_selector_1/25 -> UnitConverter_36/1  "<VINP_RemainChrgTime_min>"
  UnitConverter_36/1 -> bus_creator/36  "VINP_RemainChrgTime_min"
  bus_selector_1/26 -> UnitConverter_37/1  "<VINP_CellTempAvg_C>"
  UnitConverter_37/1 -> bus_creator/37  "VINP_CellTempAvg_C"
  bus_selector_1/27 -> UnitConverter_38/1  "<VINP_HVBCellVoltMax_mV>"
  UnitConverter_38/1 -> bus_creator/38  "VINP_HVBCellVoltMax_mV"
  bus_selector_1/28 -> UnitConverter_39/1  "<VINP_HVBCellVoltMin_mV>"
  UnitConverter_39/1 -> bus_creator/39  "VINP_HVBCellVoltMin_mV"
  bus_selector_1/29 -> UnitConverter_40/1  "<VINP_HVBMTempMax_C>"
  UnitConverter_40/1 -> bus_creator/40  "VINP_HVBMTempMax_C"
  bus_selector_1/30 -> UnitConverter_41/1  "<VINP_HVBMTempMin_C>"
  UnitConverter_41/1 -> bus_creator/41  "VINP_HVBMTempMin_C"
  bus_selector_1/31 -> UnitConverter_42/1  "<VINP_MaxCellTempNum_enum>"
  UnitConverter_42/1 -> bus_creator/42  "VINP_MaxCellTempNum_enum"
  bus_selector_1/32 -> UnitConverter_43/1  "<VINP_MaxCellVoltNum_enum>"
  UnitConverter_43/1 -> bus_creator/43  "VINP_MaxCellVoltNum_enum"
  bus_selector_1/33 -> UnitConverter_44/1  "<VINP_MinCellTempNum_enum>"
  UnitConverter_44/1 -> bus_creator/44  "VINP_MinCellTempNum_enum"
  bus_selector_1/34 -> UnitConverter_45/1  "<VINP_MinCellVoltNum_enum>"
  UnitConverter_45/1 -> bus_creator/45  "VINP_MinCellVoltNum_enum"
  bus_selector_1/35 -> UnitConverter_46/1  "<VINP_HVInVolt_V>"
  UnitConverter_46/1 -> bus_creator/46  "VINP_HVInVolt_V"
  bus_selector_1/36 -> UnitConverter_47/1  "<VINP_LVBattDet12V_V>"
  UnitConverter_47/1 -> bus_creator/47  "VINP_LVBattDet12V_V"
  bus_selector_1/37 -> UnitConverter_48/1  "<VINP_OBCDCCurLm_A>"
  UnitConverter_48/1 -> bus_creator/48  "VINP_OBCDCCurLm_A"
  bus_selector_1/38 -> UnitConverter_49/1  "<VINP_OBCDCVoltLm_V>"
  UnitConverter_49/1 -> bus_creator/49  "VINP_OBCDCVoltLm_V"
  bus_selector_1/39 -> UnitConverter_50/1  "<VINP_BMSChckSum_enum>"
  UnitConverter_50/1 -> bus_creator/50  "VINP_BMSChckSum_enum"
  bus_selector_1/40 -> UnitConverter_51/1  "<VINP_BMSRolCnct_enum>"
  UnitConverter_51/1 -> bus_creator/51  "VINP_BMSRolCnct_enum"
  bus_selector_1/41 -> UnitConverter_52/1  "<VINP_BMSREADY_flg>"
  UnitConverter_52/1 -> bus_creator/52  "VINP_BMSREADY_flg"
  bus_selector_1/42 -> UnitConverter_53/1  "<VINP_BMSWarn1_flg>"
  UnitConverter_53/1 -> bus_creator/53  "VINP_BMSWarn1_flg"
  bus_selector_1/43 -> UnitConverter_54/1  "<VINP_BMSWarn2_flg>"
  UnitConverter_54/1 -> bus_creator/54  "VINP_BMSWarn2_flg"
  bus_selector_1/44 -> UnitConverter_55/1  "<VINP_BMSWarn3_flg>"
  UnitConverter_55/1 -> bus_creator/55  "VINP_BMSWarn3_flg"
  bus_selector_1/45 -> UnitConverter_56/1  "<VINP_BMSWarn4_flg>"
  UnitConverter_56/1 -> bus_creator/56  "VINP_BMSWarn4_flg"
  bus_selector_1/46 -> UnitConverter_57/1  "<VINP_BMSWarn5_flg>"
  UnitConverter_57/1 -> bus_creator/57  "VINP_BMSWarn5_flg"
  bus_selector_1/47 -> UnitConverter_58/1  "<VINP_BMSWarn6_flg>"
  UnitConverter_58/1 -> bus_creator/58  "VINP_BMSWarn6_flg"
  bus_selector_1/48 -> UnitConverter_59/1  "<VINP_BMSWarn7_flg>"
  UnitConverter_59/1 -> bus_creator/59  "VINP_BMSWarn7_flg"
  bus_selector_1/49 -> UnitConverter_60/1  "<VINP_BMSWarn8_flg>"
  UnitConverter_60/1 -> bus_creator/60  "VINP_BMSWarn8_flg"
  bus_selector_1/50 -> UnitConverter_61/1  "<VINP_ChrgPlugSta_enum>"
  UnitConverter_61/1 -> bus_creator/61  "VINP_ChrgPlugSta_enum"
  bus_selector_1/51 -> UnitConverter_62/1  "<VINP_DisChrgPlugErr_enum>"
  UnitConverter_62/1 -> bus_creator/62  "VINP_DisChrgPlugErr_enum"
  bus_selector_1/52 -> UnitConverter_63/1  "<VINP_ExtChrgSta_enum>"
  UnitConverter_63/1 -> bus_creator/63  "VINP_ExtChrgSta_enum"
  bus_selector_1/53 -> UnitConverter_64/1  "<VINP_HVBChrgErr_enum>"
  UnitConverter_64/1 -> bus_creator/64  "VINP_HVBChrgErr_enum"
  bus_selector_1/54 -> UnitConverter_65/1  "<VINP_HVBContactorSta_flg>"
  UnitConverter_65/1 -> bus_creator/65  "VINP_HVBContactorSta_flg"
  bus_selector_1/55 -> UnitConverter_66/1  "<VINP_HVBHVILErr_flg>"
  UnitConverter_66/1 -> bus_creator/66  "VINP_HVBHVILErr_flg"
  bus_selector_1/56 -> UnitConverter_67/1  "<VINP_HVBOvrTempErr_flg>"
  UnitConverter_67/1 -> bus_creator/67  "VINP_HVBOvrTempErr_flg"
  bus_selector_1/57 -> UnitConverter_68/1  "<VINP_HVBOvrTempWarn_enum>"
  UnitConverter_68/1 -> bus_creator/68  "VINP_HVBOvrTempWarn_enum"
  bus_selector_1/58 -> UnitConverter_69/1  "<VINP_HVBPreheatPrecoolSta_enum>"
  UnitConverter_69/1 -> bus_creator/69  "VINP_HVBPreheatPrecoolSta_enum"
  bus_selector_1/59 -> UnitConverter_70/1  "<VINP_HVBattReady4Pre_enum>"
  UnitConverter_70/1 -> bus_creator/70  "VINP_HVBattReady4Pre_enum"
  bus_selector_1/60 -> UnitConverter_71/1  "<VINP_HVILSta_flg>"
  UnitConverter_71/1 -> bus_creator/71  "VINP_HVILSta_flg"
  bus_selector_1/61 -> UnitConverter_72/1  "<VINP_V2LSta_enum>"
  UnitConverter_72/1 -> bus_creator/72  "VINP_V2LSta_enum"
  bus_selector_1/62 -> UnitConverter_73/1  "<VINP_MainRlyNegSta_enum>"
  UnitConverter_73/1 -> bus_creator/73  "VINP_MainRlyNegSta_enum"
  bus_selector_1/63 -> UnitConverter_74/1  "<VINP_MainRlyPosSta_enum>"
  UnitConverter_74/1 -> bus_creator/74  "VINP_MainRlyPosSta_enum"
  bus_selector_1/64 -> UnitConverter_75/1  "<VINP_CSCCU1_enum>"
  UnitConverter_75/1 -> bus_creator/75  "VINP_CSCCU1_enum"
  bus_selector_1/65 -> UnitConverter_76/1  "<VINP_DCDCAuxCur_A>"
  UnitConverter_76/1 -> bus_creator/76  "VINP_DCDCAuxCur_A"
  bus_selector_1/66 -> UnitConverter_77/1  "<VINP_DCDCAuxVolt_V>"
  UnitConverter_77/1 -> bus_creator/77  "VINP_DCDCAuxVolt_V"
  bus_selector_1/67 -> UnitConverter_78/1  "<VINP_DCDCHVCur_A>"
  UnitConverter_78/1 -> bus_creator/78  "VINP_DCDCHVCur_A"
  bus_selector_1/68 -> UnitConverter_79/1  "<VINP_DCDCInVoltInf_V>"
  UnitConverter_79/1 -> bus_creator/79  "VINP_DCDCInVoltInf_V"
  bus_selector_1/69 -> UnitConverter_80/1  "<VINP_DCDCPreCompleted_enum>"
  UnitConverter_80/1 -> bus_creator/80  "VINP_DCDCPreCompleted_enum"
  bus_selector_1/70 -> UnitConverter_81/1  "<VINP_OBCDCCurrInf_A>"
  UnitConverter_81/1 -> bus_creator/81  "VINP_OBCDCCurrInf_A"
  bus_selector_1/71 -> UnitConverter_82/1  "<VINP_OBCDCVoltInf_V>"
  UnitConverter_82/1 -> bus_creator/82  "VINP_OBCDCVoltInf_V"
  bus_selector_1/72 -> UnitConverter_83/1  "<VINP_OBCPreCompleted_enum>"
  UnitConverter_83/1 -> bus_creator/83  "VINP_OBCPreCompleted_enum"
  bus_selector_1/73 -> UnitConverter_84/1  "<VINP_OBCWakeup4Plugin_flg>"
  UnitConverter_84/1 -> bus_creator/84  "VINP_OBCWakeup4Plugin_flg"
  bus_selector_1/74 -> UnitConverter_85/1  "<VINP_RCCCU1_enum>"
  UnitConverter_85/1 -> bus_creator/85  "VINP_RCCCU1_enum"
  bus_selector_1/75 -> UnitConverter_86/1  "<VINP_CSCCU2_enum>"
  UnitConverter_86/1 -> bus_creator/86  "VINP_CSCCU2_enum"
  bus_selector_1/76 -> UnitConverter_87/1  "<VINP_DCDCEnaSta_flg>"
  UnitConverter_87/1 -> bus_creator/87  "VINP_DCDCEnaSta_flg"
  bus_selector_1/77 -> UnitConverter_88/1  "<VINP_DCDCFaultSta_enum>"
  UnitConverter_88/1 -> bus_creator/88  "VINP_DCDCFaultSta_enum"
  bus_selector_1/78 -> UnitConverter_89/1  "<VINP_DCDCReady4Pre_flg>"
  UnitConverter_89/1 -> bus_creator/89  "VINP_DCDCReady4Pre_flg"
  bus_selector_1/79 -> UnitConverter_90/1  "<VINP_DCDCTemp_C>"
  UnitConverter_90/1 -> bus_creator/90  "VINP_DCDCTemp_C"
  bus_selector_1/80 -> UnitConverter_91/1  "<VINP_OBCACCurrInf_A>"
  UnitConverter_91/1 -> bus_creator/91  "VINP_OBCACCurrInf_A"
  bus_selector_1/81 -> UnitConverter_92/1  "<VINP_OBCACVoltInf_V>"
  UnitConverter_92/1 -> bus_creator/92  "VINP_OBCACVoltInf_V"
  bus_selector_1/82 -> UnitConverter_93/1  "<VINP_OBCEnaSta_flg>"
  UnitConverter_93/1 -> bus_creator/93  "VINP_OBCEnaSta_flg"
  bus_selector_1/83 -> UnitConverter_94/1  "<VINP_OBCFaultSta_enum>"
  UnitConverter_94/1 -> bus_creator/94  "VINP_OBCFaultSta_enum"
  bus_selector_1/84 -> UnitConverter_95/1  "<VINP_OBCPluginSta_flg>"
  UnitConverter_95/1 -> bus_creator/95  "VINP_OBCPluginSta_flg"
  bus_selector_1/85 -> UnitConverter_96/1  "<VINP_OBCReady4Pre_flg>"
  UnitConverter_96/1 -> bus_creator/96  "VINP_OBCReady4Pre_flg"
  bus_selector_1/86 -> UnitConverter_97/1  "<VINP_OBCTemp_C>"
  UnitConverter_97/1 -> bus_creator/97  "VINP_OBCTemp_C"
  bus_selector_1/87 -> UnitConverter_98/1  "<VINP_OBCV2LSta_enum>"
  UnitConverter_98/1 -> bus_creator/98  "VINP_OBCV2LSta_enum"
  bus_selector_1/88 -> UnitConverter_99/1  "<VINP_OBCACCurLim_enum>"
  UnitConverter_99/1 -> bus_creator/99  "VINP_OBCACCurLim_enum"
  bus_selector_1/89 -> UnitConverter_100/1  "<VINP_RCCCU2_enum>"
  UnitConverter_100/1 -> bus_creator/100  "VINP_RCCCU2_enum"
  bus_selector_1/90 -> UnitConverter_101/1  "<VINP_MCUWarnR_enum>"
  UnitConverter_101/1 -> bus_creator/101  "VINP_MCUWarnR_enum"
  bus_selector_1/91 -> UnitConverter_102/1  "<VINP_RrActvDmpDisabSta_flg>"
  UnitConverter_102/1 -> bus_creator/102  "VINP_RrActvDmpDisabSta_flg"
  bus_selector_1/92 -> UnitConverter_103/1  "<VINP_RrEDUDrtSta_flg>"
  UnitConverter_103/1 -> bus_creator/103  "VINP_RrEDUDrtSta_flg"
  bus_selector_1/93 -> UnitConverter_104/1  "<VINP_RrEDUOpratingSta_flg>"
  UnitConverter_104/1 -> bus_creator/104  "VINP_RrEDUOpratingSta_flg"
  bus_selector_1/94 -> UnitConverter_105/1  "<VINP_RrEDURealTMTq_Nm>"
  UnitConverter_105/1 -> bus_creator/105  "VINP_RrEDURealTMTq_Nm"
  bus_selector_1/95 -> UnitConverter_106/1  "<VINP_RrEDURotateDirction_enum>"
  UnitConverter_106/1 -> bus_creator/106  "VINP_RrEDURotateDirction_enum"
  bus_selector_1/96 -> UnitConverter_107/1  "<VINP_RrEDUTqReqFbk_Nm>"
  UnitConverter_107/1 -> bus_creator/107  "VINP_RrEDUTqReqFbk_Nm"
  bus_selector_1/97 -> UnitConverter_108/1  "<VINP_RrMCUBAT_V>"
  UnitConverter_108/1 -> bus_creator/108  "VINP_RrMCUBAT_V"
  bus_selector_1/98 -> UnitConverter_109/1  "<VINP_RrMCUDCBusCurr_A>"
  UnitConverter_109/1 -> bus_creator/109  "VINP_RrMCUDCBusCurr_A"
  bus_selector_1/99 -> UnitConverter_110/1  "<VINP_RrMCUDCBusVolt_V>"
  UnitConverter_110/1 -> bus_creator/110  "VINP_RrMCUDCBusVolt_V"
  bus_selector_1/100 -> UnitConverter_111/1  "<VINP_RrMCUDischrgSta_flg>"
  UnitConverter_111/1 -> bus_creator/111  "VINP_RrMCUDischrgSta_flg"
  bus_selector_1/101 -> UnitConverter_112/1  "<VINP_RrMCUEnaSta_flg>"
  UnitConverter_112/1 -> bus_creator/112  "VINP_RrMCUEnaSta_flg"
  bus_selector_1/102 -> UnitConverter_113/1  "<VINP_RrMCUErr_enum>"
  UnitConverter_113/1 -> bus_creator/113  "VINP_RrMCUErr_enum"
  bus_selector_1/103 -> UnitConverter_114/1  "<VINP_RrMCUIGNsta_flg>"
  UnitConverter_114/1 -> bus_creator/114  "VINP_RrMCUIGNsta_flg"
  bus_selector_1/104 -> UnitConverter_115/1  "<VINP_RrMCUReady_flg>"
  UnitConverter_115/1 -> bus_creator/115  "VINP_RrMCUReady_flg"
  bus_selector_1/105 -> UnitConverter_116/1  "<VINP_RrMCUReady4Pre_flg>"
  UnitConverter_116/1 -> bus_creator/116  "VINP_RrMCUReady4Pre_flg"
  bus_selector_1/106 -> UnitConverter_117/1  "<VINP_RrMCUSysSta_enum>"
  UnitConverter_117/1 -> bus_creator/117  "VINP_RrMCUSysSta_enum"
  bus_selector_1/107 -> UnitConverter_118/1  "<VINP_RrMCUTemp_C>"
  UnitConverter_118/1 -> bus_creator/118  "VINP_RrMCUTemp_C"
  bus_selector_1/108 -> UnitConverter_119/1  "<VINP_RrMotorAvailTq_Nm>"
  UnitConverter_119/1 -> bus_creator/119  "VINP_RrMotorAvailTq_Nm"
  bus_selector_1/109 -> UnitConverter_120/1  "<VINP_RrRegenAvailTq_Nm>"
  UnitConverter_120/1 -> bus_creator/120  "VINP_RrRegenAvailTq_Nm"
  bus_selector_1/110 -> UnitConverter_121/1  "<VINP_RrTMSpd_rpm>"
  UnitConverter_121/1 -> bus_creator/121  "VINP_RrTMSpd_rpm"
  bus_selector_1/111 -> UnitConverter_122/1  "<VINP_RrTMTemp_C>"
  UnitConverter_122/1 -> bus_creator/122  "VINP_RrTMTemp_C"
  bus_selector_1/112 -> UnitConverter_123/1  "<VINP_RrTMid_A>"
  UnitConverter_123/1 -> bus_creator/123  "VINP_RrTMid_A"
  bus_selector_1/113 -> UnitConverter_124/1  "<VINP_RrTMiq_A>"
  UnitConverter_124/1 -> bus_creator/124  "VINP_RrTMiq_A"
  bus_selector_1/114 -> UnitConverter_125/1  "<VINP_RrCoolanttempReq_cnt>"
  UnitConverter_125/1 -> bus_creator/125  "VINP_RrCoolanttempReq_cnt"
  bus_selector_1/115 -> UnitConverter_126/1  "<VINP_RrFailcode1_enum>"
  UnitConverter_126/1 -> bus_creator/126  "VINP_RrFailcode1_enum"
  bus_selector_1/116 -> UnitConverter_127/1  "<VINP_RrFailcode2_enum>"
  UnitConverter_127/1 -> bus_creator/127  "VINP_RrFailcode2_enum"
  bus_selector_1/117 -> UnitConverter_128/1  "<VINP_RrFailcodehistory1_enum>"
  UnitConverter_128/1 -> bus_creator/128  "VINP_RrFailcodehistory1_enum"
  bus_selector_1/118 -> UnitConverter_129/1  "<VINP_RrFailcodehistory2_enum>"
  UnitConverter_129/1 -> bus_creator/129  "VINP_RrFailcodehistory2_enum"
  bus_selector_1/119 -> UnitConverter_130/1  "<VINP_RrLLCTemp_C>"
  UnitConverter_130/1 -> bus_creator/130  "VINP_RrLLCTemp_C"
  bus_selector_1/120 -> UnitConverter_131/1  "<VINP_RrLLCflowReq_Lpmin>"
  UnitConverter_131/1 -> bus_creator/131  "VINP_RrLLCflowReq_Lpmin"
  bus_selector_1/121 -> UnitConverter_132/1  "<VINP_RrMCU3HWVer_enum>"
  UnitConverter_132/1 -> bus_creator/132  "VINP_RrMCU3HWVer_enum"
  bus_selector_1/122 -> UnitConverter_133/1  "<VINP_RrMCU3SWVer_enum>"
  UnitConverter_133/1 -> bus_creator/133  "VINP_RrMCU3SWVer_enum"
  bus_selector_1/123 -> UnitConverter_134/1  "<VINP_RrMCUTempWarn_enum>"
  UnitConverter_134/1 -> bus_creator/134  "VINP_RrMCUTempWarn_enum"
  bus_selector_1/124 -> UnitConverter_135/1  "<VINP_RrTMTempWarn_enum>"
  UnitConverter_135/1 -> bus_creator/135  "VINP_RrTMTempWarn_enum"
  bus_selector_1/125 -> UnitConverter_136/1  "<VINP_ShifterCRC8_enum>"
  UnitConverter_136/1 -> bus_creator/136  "VINP_ShifterCRC8_enum"
  bus_selector_1/126 -> UnitConverter_137/1  "<VINP_ShifterFailsta_enum>"
  UnitConverter_137/1 -> bus_creator/137  "VINP_ShifterFailsta_enum"
  bus_selector_1/127 -> UnitConverter_138/1  "<VINP_ShifterHandleCmd_enum>"
  UnitConverter_138/1 -> bus_creator/138  "VINP_ShifterHandleCmd_enum"
  bus_selector_1/128 -> UnitConverter_139/1  "<VINP_ShifterRC_enum>"
  UnitConverter_139/1 -> bus_creator/139  "VINP_ShifterRC_enum"
  [inp_CanValid_bus] -> bus_selector/1
  [inp_Hal_bus] -> bus_selector_1/1
  bus_creator/1 -> BINP_outputs/1
